simulink model "wide_power_acc_tb"  (R2012b)
(part 4 of 4)

      | <p style=" margin-top:0px; margin-bottom:0px; margin-left:0px; margin-right:0px; -qt-block-indent:0; text-indent:0px;"><img src="/home/observer/tools/Xilinx/14.5/ISE_DS/ISE/sysgen/data/images/xbip_dsp48_macro_v2_1_regimag.png" /></p></body></html>
      settings: infoedit=<html>Valid operands: CONCAT, P, C, PCIN, P>>17, PCIN>>17, CARRYIN, CARRYCASCIN, ACIN, A, BCIN,B<br><br>Valid operators: +, -, *, ()<br><br>Valid functions: RNDSIMPLE, RNDSYM<br><br>Instructions are case insensitive and tolerate spaces.</html>
  p : Outport
  wires:
  third/1 -> Terminator1/1
  BitBasher/1 -> p/1
  fourth/1 -> BitBasher/1
  Delay2/1 -> fourth/2, fourth/1
  Delay1/1 -> third/2, third/1
  b/1 -> Delay1/1
  a/1 -> Delay2/1
  third/2 -> fourth/3
  Delay/1 -> second/2, second/1
  c/1 -> Delay/1
  d/1 -> first/2, first/1
  first/1 -> Terminator2/1
  second/2 -> third/3
  second/1 -> Terminator/1
  first/2 -> second/3
